simulink model "tanksSMCkalman"  (R2023b)
settings: Solver=VariableStepAuto  StartTime=0.0  StopTime=150  RelTol=1e-3
values from neighbouring files (symbols this model uses):
  a1 = 0.145    [main.m]
  a2 = 0.150    (= 0.15)    [main.m]
  A_a = 35    [main.m]
  fh = [3 4 5 6 7 8 9 10 11 12 13 14 15]    [main.m]
  fq = [17.75 21.65 23.76 27.55 30.01 31.98 33.88 38.18 46.28 49.88]    [main.m]
  fu = [0.5 1 1.5 2 2.5 3 3.5 5 8 10]    [main.m]
  fv = [0.909 1.685 2.475 3.255 4.055 4.804 5.573 6.332 7.121 7.847 8.617 9.405 10.18]    [main.m]
  h0 = 3.2    [main.m]
  h10 = 7.5    [main.m]
  N = eye(2)    [main.m]
  P0 = zeros(2)    [main.m]
  Q = 0.01*eye(2)    [main.m]
  R = Np    (= 0.0001)    [main.m]
  Ts = 0.05    [main.m]
  u0 = 1    [main.m]
  x0 = [-8 -8]'    [main.m]
undefined symbols (not defined in the file or in its folder): Ad, Bd, Cd
libraries: simulink x3
settings Model: Creator=vickay-0  LastModifiedBy=virry

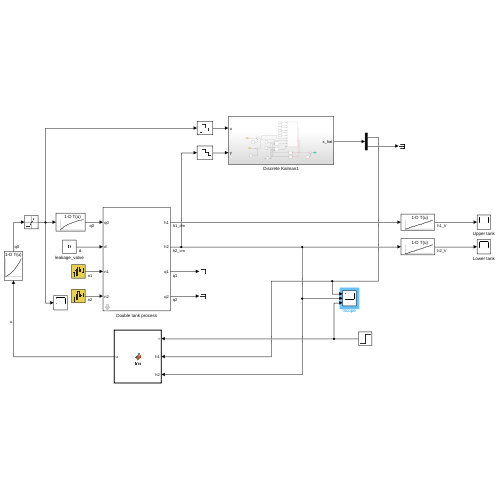
[thumbnail: Simulink's stored preview of the top-level diagram]
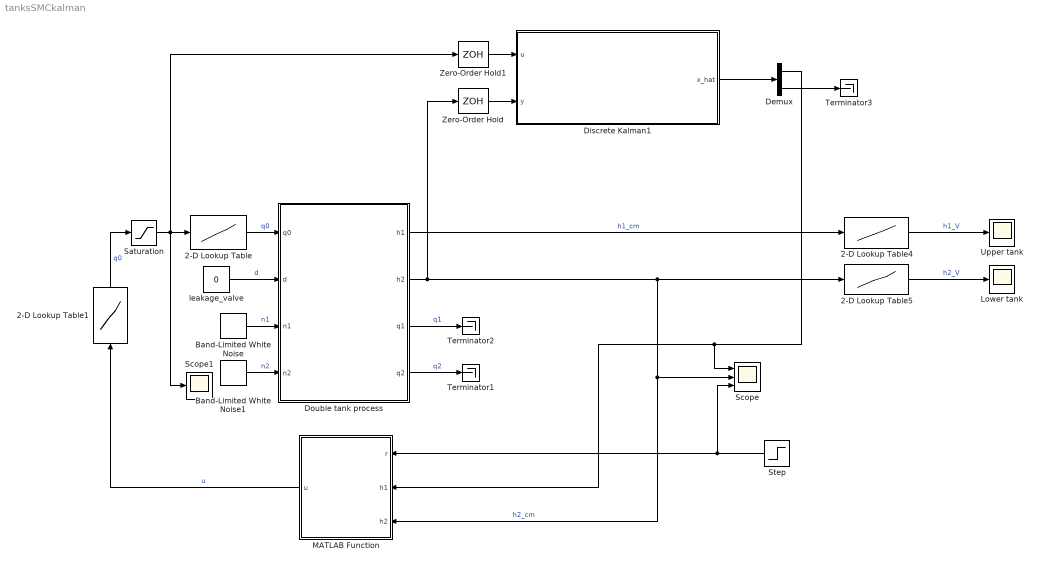
== system tanksSMCkalman ==
  2-D Lookup Table : Lookup_n-D  NumberOfTableDimensions=1  BreakpointsForDimension1=x  BreakpointsForDimension2=[1:3]  Table=y  RndMeth=Simplest  mask{x=fu, y=fq}
      mask prompts: x "Values on x-axis"; y "Values on y-axis"
  2-D Lookup Table1 : Lookup_n-D  NumberOfTableDimensions=1  BreakpointsForDimension1=x  BreakpointsForDimension2=[1:3]  Table=y  RndMeth=Simplest  mask{x=fq, y=fu}
      mask prompts: x "Values on x-axis"; y "Values on y-axis"
  2-D Lookup Table4 : Lookup_n-D  NumberOfTableDimensions=1  BreakpointsForDimension1=x  BreakpointsForDimension2=[1:3]  Table=y  RndMeth=Simplest  mask{x=fh, y=fv}
      mask prompts: x "Values on x-axis"; y "Values on y-axis"
  2-D Lookup Table5 : Lookup_n-D  NumberOfTableDimensions=1  BreakpointsForDimension1=x  BreakpointsForDimension2=[1:3]  Table=y  RndMeth=Simplest  mask{x=fh, y=fv}
      mask prompts: x "Values on x-axis"; y "Values on y-axis"
  Band-Limited White Noise : simulink/Sources/Band-Limited White Noise  Cov=Np  Ts=Ts  seed=[23341]
  Band-Limited White Noise1 : simulink/Sources/Band-Limited White Noise  Cov=Np  Ts=Ts  seed=[23341]
  Demux : Demux  Outputs=2
  Discrete Kalman1 : Subsystem
  Double tank process : Subsystem  mask{At=A_a, Ao=a1, hmax=15.5}
      mask prompts: At "Tank area (cm^2)"; Ao "Opening area (cm^2)"; hmax "Tank height (cm)"
      mask help: Double tank process parameters
  Lower tank : Scope
  MATLAB Function : MATLAB Function  TreatAsAtomicUnit=on  SystemSampleTime=Ts
  Saturation : Saturate  UpperLimit=10  LowerLimit=0
  Scope : Scope  NumInputPorts=3
  Scope1 : Scope
  Step : Step  Time=0  After=5  SampleTime=0
  Terminator1 : Terminator
  Terminator2 : Terminator
  Terminator3 : Terminator
  Upper tank : Scope
  Zero-Order Hold : ZeroOrderHold  SampleTime=Ts
  Zero-Order Hold1 : ZeroOrderHold  SampleTime=Ts
  leakage_valve : Constant  Value=0
  wires:
  2-D Lookup Table5/1 -> Lower tank/1  "h2_V"
  Double tank process/3(q1) -> Terminator2/1  "q1"
  2-D Lookup Table/1 -> Double tank process/1(q0)  "q0"
  2-D Lookup Table4/1 -> Upper tank/1  "h1_V"
  MATLAB Function/1(u) -> 2-D Lookup Table1/1  "u"
  Double tank process/4(q2) -> Terminator1/1  "q2"
  leakage_valve/1 -> Double tank process/2(d)  "d"
  Double tank process/2(h2) -> Scope/2, MATLAB Function/3(h2), 2-D Lookup Table5/1, Zero-Order Hold/1  "h2_cm"
  Double tank process/1(h1) -> 2-D Lookup Table4/1  "h1_cm"
  Step/1 -> Scope/3, MATLAB Function/1(r)
  2-D Lookup Table1/1 -> Saturation/1  "q0"
  Saturation/1 -> Zero-Order Hold1/1, Scope1/1, 2-D Lookup Table/1
  Discrete Kalman1/1(x_hat) -> Demux/1
  Demux/1 -> MATLAB Function/2(h1), Scope/1
  Zero-Order Hold/1 -> Discrete Kalman1/2(y)
  Zero-Order Hold1/1 -> Discrete Kalman1/1(u)
  Band-Limited White Noise/1 -> Double tank process/3(n1)  "n1"
  Band-Limited White Noise1/1 -> Double tank process/4(n2)  "n2"
  Demux/2 -> Terminator3/1

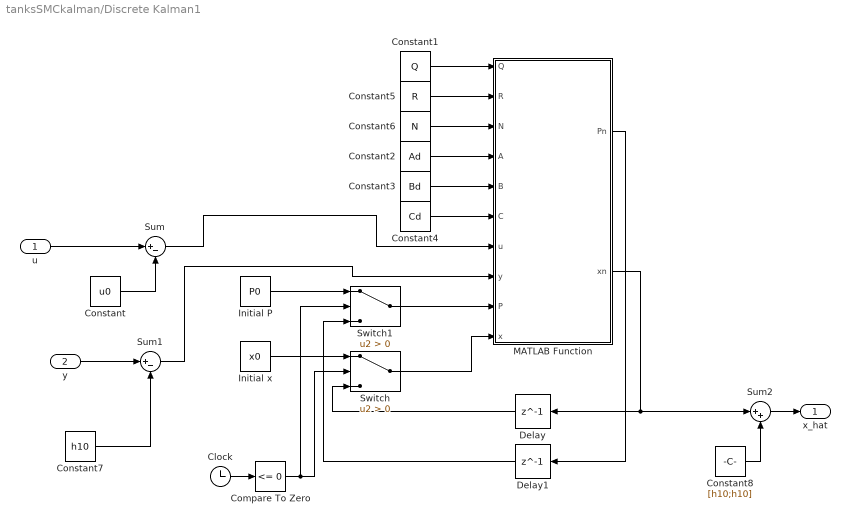
== system tanksSMCkalman/Discrete Kalman1 ==
  u : Inport  OutDataTypeStr=double  PortDimensions=1
  y : Inport  Port=2  OutDataTypeStr=double  PortDimensions=1
  Clock : Clock
  Compare To Zero : simulink/Logic and Bit Operations/Compare To Zero  relop=<=  OutDataTypeStr=boolean
  Constant : Constant  Value=u0
  Constant1 : Constant  Value=Q  VectorParams1D=off
  Constant2 : Constant  Value=Ad  VectorParams1D=off
  Constant3 : Constant  Value=Bd  VectorParams1D=off
  Constant4 : Constant  Value=Cd  VectorParams1D=off
  Constant5 : Constant  Value=R  VectorParams1D=off
  Constant6 : Constant  Value=N  VectorParams1D=off
  Constant7 : Constant  Value=h10
  Constant8 : Constant  Value=[h10;h10]
  Delay : Delay  DelayLength=1  InitialCondition=0  SampleTime=Ts
  Delay1 : Delay  DelayLength=1  InitialCondition=0  SampleTime=Ts
  Initial P : Constant  Value=P0
  Initial x : Constant  Value=x0
  MATLAB Function : MATLAB Function  TreatAsAtomicUnit=on  SystemSampleTime=Ts
  Sum : Sum  Inputs=|+-
  Sum1 : Sum  Inputs=|+-
  Sum2 : Sum  Inputs=|++
  Switch : Switch  Criteria=u2 > Threshold  SaturateOnIntegerOverflow=off  InputSameDT=off
  Switch1 : Switch  Criteria=u2 > Threshold  SaturateOnIntegerOverflow=off  InputSameDT=off
  x_hat : Outport
  wires:
  Clock/1 -> Compare To Zero/1
  Initial x/1 -> Switch/1
  Compare To Zero/1 -> Switch/2, Switch1/2
  Switch1/1 -> MATLAB Function/9(P)
  Initial P/1 -> Switch1/1
  Delay1/1 -> Switch1/3
  Delay/1 -> Switch/3
  Switch/1 -> MATLAB Function/10(x)
  MATLAB Function/1(Pn) -> Delay1/1
  MATLAB Function/2(xn) -> Delay/1, Sum2/1
  Sum1/1 -> MATLAB Function/8(y)
  Sum/1 -> MATLAB Function/7(u)
  Constant4/1 -> MATLAB Function/6(C)
  Constant3/1 -> MATLAB Function/5(B)
  Constant2/1 -> MATLAB Function/4(A)
  Constant6/1 -> MATLAB Function/3(N)
  Constant5/1 -> MATLAB Function/2(R)
  Constant1/1 -> MATLAB Function/1(Q)
  u/1 -> Sum/1
  Constant/1 -> Sum/2
  Constant7/1 -> Sum1/2
  y/1 -> Sum1/1
  Constant8/1 -> Sum2/2
  Sum2/1 -> x_hat/1

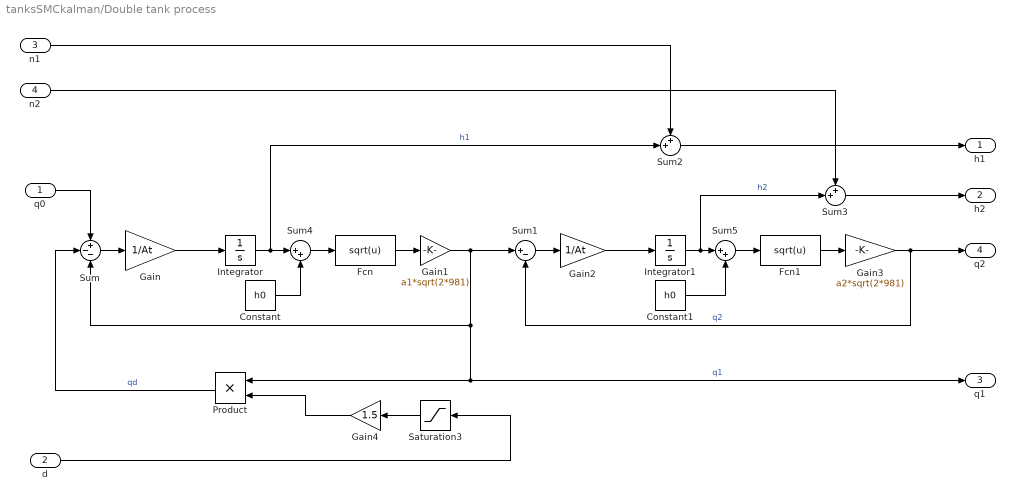
== system tanksSMCkalman/Double tank process ==
  q0 : Inport
  d : Inport  Port=2
  n1 : Inport  Port=3
  n2 : Inport  Port=4
  Constant : Constant  Value=h0
  Constant1 : Constant  Value=h0
  Fcn : Fcn  Expr=sqrt(u)
  Fcn1 : Fcn  Expr=sqrt(u)
  Gain : Gain  Gain=1/At
  Gain1 : Gain  Gain=a1*sqrt(2*981)
  Gain2 : Gain  Gain=1/At
  Gain3 : Gain  Gain=a2*sqrt(2*981)
  Gain4 : Gain  Gain=1.5
  Integrator : Integrator  LimitOutput=on  UpperSaturationLimit=hmax  LowerSaturationLimit=0
  Integrator1 : Integrator  LimitOutput=on  UpperSaturationLimit=hmax  LowerSaturationLimit=0
  Product : Product  RndMeth=Zero
  Saturation3 : Saturate  UpperLimit=1  LowerLimit=0
  Sum : Sum  Inputs=+--
  Sum1 : Sum  Inputs=|+-
  Sum2 : Sum  Inputs=++|
  Sum3 : Sum  Inputs=++|
  Sum4 : Sum  Inputs=|++
  Sum5 : Sum  Inputs=|++
  h1 : Outport  VectorParamsAs1DForOutWhenUnconnected=off
  h2 : Outport  Port=2  VectorParamsAs1DForOutWhenUnconnected=off
  q1 : Outport  Port=3  VectorParamsAs1DForOutWhenUnconnected=off
  q2 : Outport  Port=4  VectorParamsAs1DForOutWhenUnconnected=off
  wires:
  Sum/1 -> Gain/1
  Gain/1 -> Integrator/1
  Fcn/1 -> Gain1/1
  Gain1/1 -> Sum1/1, Product/1, q1/1, Sum/3  "q1"
  Sum1/1 -> Gain2/1
  Gain2/1 -> Integrator1/1
  Fcn1/1 -> Gain3/1
  Gain3/1 -> Sum1/2, q2/1  "q2"
  q0/1 -> Sum/1
  Integrator/1 -> Sum4/1, Sum2/2  "h1"
  Product/1 -> Sum/2  "qd"
  d/1 -> Saturation3/1
  Integrator1/1 -> Sum5/1, Sum3/2  "h2"
  Saturation3/1 -> Gain4/1
  Gain4/1 -> Product/2
  Sum2/1 -> h1/1
  n1/1 -> Sum2/1
  Sum3/1 -> h2/1
  n2/1 -> Sum3/1
  Sum4/1 -> Fcn/1
  Constant/1 -> Sum4/2
  Sum5/1 -> Fcn1/1
  Constant1/1 -> Sum5/2

== matlab function tanksSMCkalman/MATLAB Function ==
  data: r input; h1 input; h2 input; u output
function u = fcn(r,h1,h2)

A = 35;   % Tank cross section
a1 = 0.145;   % Outlet cross section
a2 = 0.155;
g = 981;    % Gravity
h0 = 3.2; 

alpha =- (a1^2*g)/A^2 - (sqrt( (2))*a2*g*((sqrt( (2))*a1*sqrt(g*(h0 + h1)))/A - (sqrt( (2))*a2*sqrt(g*(h0 + h2)))/A))/(2*A*sqrt(g*(h0 + h2)));
beta = (sqrt( (2))*a1*g)/(2*A^2*sqrt(g*(h0 + h1)));
h2_dot = (sqrt(2)*a1*sqrt(g*(h0 + h1)))/A - (sqrt(2)*a2*sqrt(g*(h0 + h2)))/A;

p = [10; 1];
mu = 20;

fx =[ alpha; h2_dot ];

gx = [beta; 0];
sigma = p'*[h2_dot (h2-r)]';

epsilon = 0.8;

if abs(sigma) < epsilon
    sat = sigma/epsilon;
else
    sat = sign(sigma);
end

u = -p'*fx/(p'*gx)-mu/(p'*gx)*sat;
u = u;

end

== matlab function tanksSMCkalman/Discrete Kalman1/MATLAB Function ==
  data: Q input; R input; N input; A input; B input; C input; u input; y input; P input; x input; Pn output; xn output
function [Pn,xn] = fcn(Q,R,N,A,B,C,u,y,P,x)

xn = [0 0]';
Pn = zeros(2);

% Predict 
xn = A * x + B * u; 
Pn = A * P * A' + N*Q*N';

% Update 
K = (Pn * C') / (C * Pn * C' + R); 
xn = xn + K * (y - C * xn); 
Pn = Pn - K*C*Pn;

end
